simulink model "Cascade_Tank"  (R2018b)
settings: Solver=ode45  StartTime=0.0  StopTime=500  RelTol=1e-3  EnableMultiTasking=on
settings Model: Creator=DUYLINH  LastModifiedBy=daiba
settings DataIOCC: LimitDataPoints=on  SaveFormat=Array
settings OptimizationCC: LifeSpan=inf
settings DebuggingCC: SFUnexpectedBacktrackingDiag=warning  SFNoUnconditionalDefaultTransitionDiag=warning  SFExecutionAtInitializationDiag=none
settings HardwareCC: ProdBitPerPointer=32  ProdBitPerSizeT=32  ProdBitPerPtrDiffT=32  ProdLargestAtomicFloat=None  ProdIntDivRoundTo=Undefined  ProdEndianess=Unspecified  ProdWordSize=32  ProdHWDeviceType=32-bit Generic
settings ModelReferenceCC: PropagateSignalLabelsOutOfModel=off
settings SFSimCC: SimUseLocalCustomCode=off
settings RTWCC: RTWUseLocalCustomCode=off
settings CodeAppCC: StateflowObjectComments=on
settings GRTTargetCC: TargetLangStandard=C89/C90 (ANSI)  GeneratePreprocessorConditionals=Disable all
settings ConfigComp: CovMetricSettings=dw  CovHtmlReporting=on  CovSaveCumulativeToWorkspaceVar=on  CovSaveSingleToWorkspaceVar=on  CovExternalEMLEnable=off

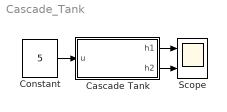
== system Cascade_Tank ==
  " Cascade Tank" : Subsystem  mask{AA=15, AAA=10, a=0.4, aaaa=0.5, k=0.2, Cd=0.6, g=9.81, h1_zero=1.5, h2_zero=1}
      mask prompts: AA "Tiet dien ngang bon chua 1"; AAA "Tiet dien ngang bon chua 2"; a "Tiet dien van xa 1"; aaaa "Tiet dien van xa 2"; k "He so ti le cong suat may bom"; Cd "He so xa"; g "Gia toc trong truong"; h1_zero "Muc nuoc ban dau bon 1"; h2_zero "Muc nuoc ban dau bon 2"
  Constant : Constant  Value=5
  Scope : Scope  NumInputPorts=2
  wires:
  " Cascade Tank"/1(h1) -> Scope/1
  Constant/1 -> " Cascade Tank"/1(u)
  " Cascade Tank"/2(h2) -> Scope/2

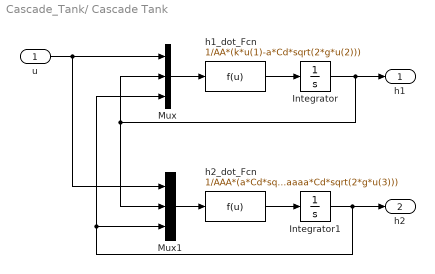
== system Cascade_Tank/ Cascade Tank ==
  u : Inport
  Integrator : Integrator  InitialCondition=h1_zero
  Integrator1 : Integrator  InitialCondition=h2_zero
  Mux : Mux  Inputs=3
  Mux1 : Mux  Inputs=3
  h1_dot_Fcn : Fcn  Expr=1/AA*(k*u(1)-a*Cd*sqrt(2*g*u(2)))
  h2_dot_Fcn : Fcn  Expr=1/AAA*(a*Cd*sqrt(2*g*u(2))-aaaa*Cd*sqrt(2*g*u(3)))
  h1 : Outport
  h2 : Outport  Port=2
  wires:
  Mux/1 -> h1_dot_Fcn/1
  h1_dot_Fcn/1 -> Integrator/1
  Integrator/1 -> Mux/2, Mux1/2, h1/1
  h2_dot_Fcn/1 -> Integrator1/1
  Mux1/1 -> h2_dot_Fcn/1
  Integrator1/1 -> Mux/3, Mux1/3, h2/1
  u/1 -> Mux1/1, Mux/1
